simulink model "adm_pcie_9h7_dts_dual_4x100g_dsp_8b_1ant"  (R2019a)
settings: Solver=VariableStepAuto  StartTime=0.0  StopTime=10.0  RelTol=1e-3
undefined symbols (not defined in the file): datetime, fft_stages, posixtime
libraries: xbsIndex_r4 x17321, casper_library_misc x181, xps_library x11, casper_library_delays x8, casper_library_sources x8, casper_library_reorder x5, casper_library_scopes x4
(part 22 of 187)

== system adm_pcie_9h7_dts_dual_4x100g_dsp_8b_1ant/pipeline0/input/bit_stats ==
  din : Inport
  Counter1 : xbsIndex_r4/Counter  cnt_type=Free Running  cnt_to=Inf  operation=Up  start_count=0  cnt_by_val=1  arith_type=Unsigned  n_bits=20  bin_pt=0  load_pin=off  rst=off  en=off  explicit_period=on  period=1  use_behavioral_HDL=off  implementation=Fabric  use_rpm=on  dbl_ovrd=off  block_type=counter
      settings: xl_area=[0, 0, 0, 0, 0, 0, 0]
  Mux : xbsIndex_r4/Mux  inputs=32  en=off  latency=1  precision=Full  arith_type=Unsigned  n_bits=16  bin_pt=14  quantization=Truncate  overflow=Wrap  dbl_ovrd=off  block_type=mux
  Slice1 : xbsIndex_r4/Slice  nbits=1  boolean_output=on  mode=Upper Bit Location + Width  bit1=0  base1=MSB of Input  bit0=19  base0=LSB of Input  dbl_ovrd=off  block_type=slice
      settings: infoedit="Extracts a given range of bits from each input sample and presents it at the output.  The output type is ordinarily unsigned with binary point at zero, but can be Boolean when the slice is one bit wide.<P><P>Hardware notes: In hardware this block costs nothing."  block_version=10.1.3
  Slice2 : xbsIndex_r4/Slice  nbits=1  boolean_output=off  mode=Lower Bit Location + Width  bit1=0  base1=MSB of Input  bit0=5  base0=LSB of Input  dbl_ovrd=off  block_type=slice
      settings: block_version=10.1.3
  Slice3 : xbsIndex_r4/Slice  nbits=5  boolean_output=off  mode=Lower Bit Location + Width  bit1=0  base1=MSB of Input  bit0=0  base0=LSB of Input  dbl_ovrd=off  block_type=slice
      settings: block_version=10.1.3
  bus_expand1 : Subsystem  AncestorBlock=casper_library_flow_control/bus_expand  mask(bus_expand){mode=divisions of equal size, outputNum=32, outputWidth=8, outputBinaryPt=0, outputArithmeticType=0, show_format=off, outputToWorkspace=off, variablePrefix=out, outputToModelAsWell=on}
      mask prompts: outputNum "Number of outputs:"; outputWidth "Output width:"; outputBinaryPt "Output binary point position:"; outputArithmeticType "Output arithmetic type (ufix=0, fix=1, bool=2):"; show_format "Print format string?"; outputToWorkspace "Output to workspace?"; variablePrefix "Variable name prefix:"; outputToModelAsWell "Output to model as well?"
      mask help:
      | Expands a 'bus' made using a bus_create or Xilinx
      | concat block.
      | The input will be divided into the specified number
      | of outputs with the specified arithmetic types.
      | Divisions are made from most significant bit.
      mask init: same as adm_pcie_9h7_dts_dual_4x100g_dsp_8b_1ant/pipeline0/autocorr/bus_expand
      settings: AttributesFormatString=32 outputs
      mask TypeOptions mode: divisions of equal size | divisions of arbitrary size
      mask Callback mode: bus_expand_callback();
      mask Callback outputWidth: bus_expand_callback();
      mask Callback outputToWorkspace: bus_expand_callback();
  edge_detect1 : Subsystem  AncestorBlock=casper_library_misc/edge_detect  mask(edge_detect){edge=Rising, polarity=Active High, x_in=[0 0.08 0.08 0.16 0.16 0.24 0.24 0.32 0.32 0.4], y_in=[-1 -1  1  1  1  1  1  1  1  1], x_out=[0.6 0.68 0.68 0.76 0.76 0.84 0.84 0.92 0.92 1], y_out=[-1 -1  1  1 -1 -1 -1 -1 -1 -1]}
      mask prompts: edge "Edge Type"; polarity "Output Polarity"; x_in "Input X Positions"; y_in "Input Y Positions"; x_out "Output X Positions"; y_out "Output Y Positions"
      mask help: Output is active for one-cycle after each edge of the specified type (i.e. rising, falling or both).
      mask init: same as adm_pcie_9h7_dts_dual_4x100g_dsp_8b_1ant/pipeline0/corr/edge_detect
      settings: AttributesFormatString=|
      | rising edges
      | active high
      mask Help: Output is active for one-cycle after each edge of the specified type (i.e. rising, falling, or both).  Latency is zero.
      mask TypeOptions edge: Rising | Falling | Both
      mask TypeOptions polarity: Active High | Active Low
      mask Display:
      | plot(x_in_num,0.5+y_in_num*0.2);
      | plot(x_out_num,0.5+y_out_num*0.2);
  histogram : Subsystem  mask{bitwidth=8}
  input_sel : Subsystem  Tag=xps:sw_reg  AncestorBlock=xps_library/Memory/software_register  mask(swreg){io_dir=From Processor, io_delay=0, init_val=0, sample_period=1, names=reg, bitwidths=32, bin_pts=0, arith_types=0, sim_port=on, show_format=on, desc_str=|}
      mask desc_str=|
      | Input selection. The least significant 6 bits should be
      | set to ``n`` to compute the histogram for input ``n``.
      mask prompts: io_dir "I/O direction"; io_delay "I/O delay"; init_val "Initial Value"; sample_period "Sample period"; names "Bitfield names [msb...lsb]"; bitwidths "Bitfield widths"; bin_pts "Bitfield binary pts"; arith_types "Bitfield types, ufix=0, fix=1, bool=2"; sim_port "Provide sim input/output?"; show_format "Print format string?"; desc_str "Description"
      mask help: A 32-bit software-accessible register. Can be divided into bitfields of varying widths and types using the fields in the block mask.
      mask init:
      | swreg_init(gcb)
      settings: AttributesFormatString=1input:uf32.0 = 32 bits
      mask TypeOptions io_dir: To Processor | From Processor
      mask Callback io_dir:
      | mask_enables = get_param(gcb, 'MaskEnables');
      | mask_names = get_param(gcb, 'MaskNames');
      | if strcmp(get_param(gcb, 'io_dir'), 'To Processor'),
      |     mask_enables{ismember(mask_names, 'sample_period')} = 'off';
      | else
      |     mask_enables{ismember(mask_names, 'sample_period')} = 'on';
      | end
      | set_param(gcb, 'MaskEnables', mask_enables);
      mask DialogControl ParameterTabVar0 Prompt: Setup
  wires:
  [adc_hist_rst] -> histogram/2(new_acc)
  Mux/1 -> histogram/1(din)
  Counter1/1 -> Slice1/1
  Slice1/1 -> edge_detect1/1(in)
  edge_detect1/1(out) -> [adc_hist_rst]
  input_sel/1(in_reg) -> Slice3/1, Slice2/1
  Slice2/1 -> [sel_msb]
  din/1 -> bus_expand1/1(bus_in)
  Slice3/1 -> [sel_lsb]
  [sel_lsb] -> Mux/1
  bus_expand1/14(out19) -> Mux/15
  bus_expand1/7(out26) -> Mux/8
  bus_expand1/13(out20) -> Mux/14
  bus_expand1/17(out16) -> Mux/18
  bus_expand1/18(out15) -> Mux/19
  bus_expand1/11(out22) -> Mux/12
  bus_expand1/20(out13) -> Mux/21
  bus_expand1/2(out31) -> Mux/3
  bus_expand1/9(out24) -> Mux/10
  bus_expand1/3(out30) -> Mux/4
  bus_expand1/6(out27) -> Mux/7
  bus_expand1/10(out23) -> Mux/11
  bus_expand1/21(out12) -> Mux/22
  bus_expand1/16(out17) -> Mux/17
  bus_expand1/19(out14) -> Mux/20
  bus_expand1/12(out21) -> Mux/13
  bus_expand1/4(out29) -> Mux/5
  bus_expand1/1(msb_out32) -> Mux/2
  bus_expand1/15(out18) -> Mux/16
  bus_expand1/5(out28) -> Mux/6
  bus_expand1/22(out11) -> Mux/23
  bus_expand1/23(out10) -> Mux/24
  bus_expand1/24(out9) -> Mux/25
  bus_expand1/25(out8) -> Mux/26
  bus_expand1/26(out7) -> Mux/27
  bus_expand1/27(out6) -> Mux/28
  bus_expand1/28(out5) -> Mux/29
  bus_expand1/29(out4) -> Mux/30
  bus_expand1/30(out3) -> Mux/31
  bus_expand1/31(out2) -> Mux/32
  bus_expand1/32(lsb_out1) -> Mux/33
  bus_expand1/8(out25) -> Mux/9

== system adm_pcie_9h7_dts_dual_4x100g_dsp_8b_1ant/pipeline0/input/bus_mux1 ==
  sel : Inport
  d0 : Inport  Port=2
  d1 : Inport  Port=3
  d2 : Inport  Port=4
  misci : Inport  Port=5
  d_bussify : Subsystem  AncestorBlock=casper_library_flow_control/bus_create  mask(bus_create){inputNum=4}
      mask prompts: inputNum "Number of inputs:"
      mask init:
      | bus_create_init(gcb,...
      |     'inputNum', inputNum);
  dmisc : xbsIndex_r4/Delay  rst=off  infoeditControl=Selection of Reset will increase slice count due to use of real FFs and instead of SRLs  en=off  latency=1  reg_retiming=on  dbl_ovrd=off  block_type=delay
  expand0 : Subsystem  AncestorBlock=casper_library_flow_control/bus_expand  mask(bus_expand){mode=divisions of arbitrary size, outputNum=1, outputWidth=[64;64;64;64], outputBinaryPt=[0  0  0  0], outputArithmeticType=[0  0  0  0], show_format=on, outputToWorkspace=off, variablePrefix=, outputToModelAsWell=on}
      mask prompts: outputNum "Number of outputs:"; outputWidth "Output width [msb ... lsb]:"; outputBinaryPt "Output binary point position [msb ... lsb]:"; outputArithmeticType "Output arithmetic type (ufix=0, fix=1, bool=2) [msb ... lsb]:"; show_format "Print format string?"; outputToWorkspace "Output to workspace?"; variablePrefix "Variable name prefix:"; outputToModelAsWell "Output to model as well?"
      mask help:
      | Expands a 'bus' made using a bus_create or Xilinx
      | concat block.
      | The input will be divided into the specified number
      | of outputs with the specified arithmetic types.
      | Divisions are made from most significant bit.
      mask init: same as adm_pcie_9h7_dts_dual_4x100g_dsp_8b_1ant/pipeline0/autocorr/bus_expand
      settings: AttributesFormatString=4 outputs: uf64.0,uf64.0,uf64.0,uf64.0,
      mask TypeOptions mode: divisions of equal size | divisions of arbitrary size
      mask Callback mode: bus_expand_callback();
      mask Callback outputWidth: bus_expand_callback();
      mask Callback outputToWorkspace: bus_expand_callback();
  expand1 : Subsystem  AncestorBlock=casper_library_flow_control/bus_expand  mask(bus_expand){mode=divisions of arbitrary size, outputNum=1, outputWidth=[64;64;64;64], outputBinaryPt=[0  0  0  0], outputArithmeticType=[0  0  0  0], show_format=on, outputToWorkspace=off, variablePrefix=, outputToModelAsWell=on}
      mask prompts: outputNum "Number of outputs:"; outputWidth "Output width [msb ... lsb]:"; outputBinaryPt "Output binary point position [msb ... lsb]:"; outputArithmeticType "Output arithmetic type (ufix=0, fix=1, bool=2) [msb ... lsb]:"; show_format "Print format string?"; outputToWorkspace "Output to workspace?"; variablePrefix "Variable name prefix:"; outputToModelAsWell "Output to model as well?"
      mask help:
      | Expands a 'bus' made using a bus_create or Xilinx
      | concat block.
      | The input will be divided into the specified number
      | of outputs with the specified arithmetic types.
      | Divisions are made from most significant bit.
      mask init: same as adm_pcie_9h7_dts_dual_4x100g_dsp_8b_1ant/pipeline0/autocorr/bus_expand
      settings: AttributesFormatString=4 outputs: uf64.0,uf64.0,uf64.0,uf64.0,
      mask TypeOptions mode: divisions of equal size | divisions of arbitrary size
      mask Callback mode: bus_expand_callback();
      mask Callback outputWidth: bus_expand_callback();
      mask Callback outputToWorkspace: bus_expand_callback();
  expand2 : Subsystem  AncestorBlock=casper_library_flow_control/bus_expand  mask(bus_expand){mode=divisions of arbitrary size, outputNum=1, outputWidth=[64;64;64;64], outputBinaryPt=[0  0  0  0], outputArithmeticType=[0  0  0  0], show_format=on, outputToWorkspace=off, variablePrefix=, outputToModelAsWell=on}
      mask prompts: outputNum "Number of outputs:"; outputWidth "Output width [msb ... lsb]:"; outputBinaryPt "Output binary point position [msb ... lsb]:"; outputArithmeticType "Output arithmetic type (ufix=0, fix=1, bool=2) [msb ... lsb]:"; show_format "Print format string?"; outputToWorkspace "Output to workspace?"; variablePrefix "Variable name prefix:"; outputToModelAsWell "Output to model as well?"
      mask help:
      | Expands a 'bus' made using a bus_create or Xilinx
      | concat block.
      | The input will be divided into the specified number
      | of outputs with the specified arithmetic types.
      | Divisions are made from most significant bit.
      mask init: same as adm_pcie_9h7_dts_dual_4x100g_dsp_8b_1ant/pipeline0/autocorr/bus_expand
      settings: AttributesFormatString=4 outputs: uf64.0,uf64.0,uf64.0,uf64.0,
      mask TypeOptions mode: divisions of equal size | divisions of arbitrary size
      mask Callback mode: bus_expand_callback();
      mask Callback outputWidth: bus_expand_callback();
      mask Callback outputToWorkspace: bus_expand_callback();
  mux{0..3} (4 alike) : xbsIndex_r4/Mux  inputs=3  en=off  latency=1  precision=Full  arith_type=Unsigned  n_bits=16  bin_pt=14  quantization=Truncate  overflow=Wrap  dbl_ovrd=off  block_type=mux
  sel_expand : Subsystem  AncestorBlock=casper_library_flow_control/bus_expand  mask(bus_expand){mode=divisions of equal size, outputNum=4, outputWidth=2, outputBinaryPt=0, outputArithmeticType=0, show_format=on, outputToWorkspace=off, variablePrefix=, outputToModelAsWell=on}
      mask prompts: outputNum "Number of outputs:"; outputWidth "Output width:"; outputBinaryPt "Output binary point position:"; outputArithmeticType "Output arithmetic type (ufix=0, fix=1, bool=2):"; show_format "Print format string?"; outputToWorkspace "Output to workspace?"; variablePrefix "Variable name prefix:"; outputToModelAsWell "Output to model as well?"
      mask help:
      | Expands a 'bus' made using a bus_create or Xilinx
      | concat block.
      | The input will be divided into the specified number
      | of outputs with the specified arithmetic types.
      | Divisions are made from most significant bit.
      mask init: same as adm_pcie_9h7_dts_dual_4x100g_dsp_8b_1ant/pipeline0/autocorr/bus_expand
      settings: AttributesFormatString=4 outputs: uf2.0,uf2.0,uf2.0,uf2.0,
      mask TypeOptions mode: divisions of equal size | divisions of arbitrary size
      mask Callback mode: bus_expand_callback();
      mask Callback outputWidth: bus_expand_callback();
      mask Callback outputToWorkspace: bus_expand_callback();
  out : Outport
  misco : Outport  Port=2
  wires:
  sel/1 -> sel_expand/1(bus_in)
  d0/1 -> expand0/1(bus_in)
  d1/1 -> expand1/1(bus_in)
  d2/1 -> expand2/1(bus_in)
  sel_expand/1(msb_out4) -> mux0/1
  expand0/1(msb_out4) -> mux0/2
  expand1/1(msb_out4) -> mux0/3
  expand2/1(msb_out4) -> mux0/4
  sel_expand/2(out3) -> mux1/1
  expand0/2(out3) -> mux1/2
  expand1/2(out3) -> mux1/3
  expand2/2(out3) -> mux1/4
  sel_expand/3(out2) -> mux2/1
  expand0/3(out2) -> mux2/2
  expand1/3(out2) -> mux2/3
  expand2/3(out2) -> mux2/4
  sel_expand/4(lsb_out1) -> mux3/1
  expand0/4(lsb_out1) -> mux3/2
  expand1/4(lsb_out1) -> mux3/3
  expand2/4(lsb_out1) -> mux3/4
  misci/1 -> dmisc/1
  mux0/1 -> d_bussify/1(in1)
  mux1/1 -> d_bussify/2(in2)
  mux2/1 -> d_bussify/3(in3)
  mux3/1 -> d_bussify/4(in4)
  d_bussify/1(bus_out) -> out/1
  dmisc/1 -> misco/1

== system adm_pcie_9h7_dts_dual_4x100g_dsp_8b_1ant/pipeline0/input/rms ==
  note: two clocks after
      | adc_rms_rst goes high
      | the outputs are locked
  note: To provide a means for measuring the magnitude of the signals
      | coming in to each ADC channel, we have a "calc_adc_sum_sq"
      | block which uses a single multiplier, two accumulators, and two
      | regsiters to calculate the sum of 64K ADC samples and the sum
      | of squares of 64K ADC samples.  These can be used to calculate
      | the mean (aka DC offset) and standard deviation (aka RMS) of
      | the ADC inputs.
  note: The sum_sumsq values are Fix_64_0.
      | The upper 29 bits are Fix_29_0 sum of samples.
      | The lower 35 bits are UFix_35_0 sum of squares.
  note: sum,sq,sum,sq,...
  in : Inport
  Constant : Constant  Value=0
  Counter : xbsIndex_r4/Counter  cnt_type=Free Running  cnt_to=Inf  operation=Up  start_count=0  cnt_by_val=1  arith_type=Unsigned  n_bits=16  bin_pt=0  load_pin=off  rst=off  en=off  explicit_period=off  period=1  use_behavioral_HDL=off  implementation=Fabric  use_rpm=on  dbl_ovrd=off  block_type=counter
      settings: xl_area=[0, 0, 0, 0, 0, 0, 0]
  Goto Tag Visibility : GotoTagVisibility  GotoTag=adc_rms_rst
  Slice16 : xbsIndex_r4/Slice  nbits=1  boolean_output=on  mode=Upper Bit Location + Width  bit1=0  base1=MSB of Input  bit0=19  base0=LSB of Input  dbl_ovrd=off  block_type=slice
      settings: infoedit="Extracts a given range of bits from each input sample and presents it at the output.  The output type is ordinarily unsigned with binary point at zero, but can be Boolean when the slice is one bit wide.<P><P>Hardware notes: In hardware this block costs nothing."  block_version=10.1.3
  Terminator : Terminator
  bram_ctrl : Subsystem
  bus_expand : Subsystem  AncestorBlock=casper_library_flow_control/bus_expand  mask(bus_expand){mode=divisions of equal size, outputNum=32, outputWidth=8, outputBinaryPt=0, outputArithmeticType=1, show_format=off, outputToWorkspace=off, variablePrefix=out, outputToModelAsWell=on}
      mask prompts: outputNum "Number of outputs:"; outputWidth "Output width:"; outputBinaryPt "Output binary point position:"; outputArithmeticType "Output arithmetic type (ufix=0, fix=1, bool=2):"; show_format "Print format string?"; outputToWorkspace "Output to workspace?"; variablePrefix "Variable name prefix:"; outputToModelAsWell "Output to model as well?"
      mask help:
      | Expands a 'bus' made using a bus_create or Xilinx
      | concat block.
      | The input will be divided into the specified number
      | of outputs with the specified arithmetic types.
      | Divisions are made from most significant bit.
      mask init: same as adm_pcie_9h7_dts_dual_4x100g_dsp_8b_1ant/pipeline0/autocorr/bus_expand
      settings: AttributesFormatString=32 outputs
      mask TypeOptions mode: divisions of equal size | divisions of arbitrary size
      mask Callback mode: bus_expand_callback();
      mask Callback outputWidth: bus_expand_callback();
      mask Callback outputToWorkspace: bus_expand_callback();
  calc_adc_sum_sq0 : Subsystem
  calc_adc_sum_sq1 : Subsystem
  calc_adc_sum_sq10 : Subsystem
  calc_adc_sum_sq11 : Subsystem
  calc_adc_sum_sq12 : Subsystem
  calc_adc_sum_sq13 : Subsystem
  calc_adc_sum_sq14 : Subsystem
  calc_adc_sum_sq15 : Subsystem
  calc_adc_sum_sq16 : Subsystem
  calc_adc_sum_sq17 : Subsystem
  calc_adc_sum_sq18 : Subsystem
  calc_adc_sum_sq19 : Subsystem
  calc_adc_sum_sq2 : Subsystem
  calc_adc_sum_sq20 : Subsystem
  calc_adc_sum_sq21 : Subsystem
  calc_adc_sum_sq22 : Subsystem
  calc_adc_sum_sq23 : Subsystem
  calc_adc_sum_sq24 : Subsystem
  calc_adc_sum_sq25 : Subsystem
  calc_adc_sum_sq26 : Subsystem
  calc_adc_sum_sq27 : Subsystem
  calc_adc_sum_sq28 : Subsystem
  calc_adc_sum_sq29 : Subsystem
  calc_adc_sum_sq3 : Subsystem
  calc_adc_sum_sq30 : Subsystem
  calc_adc_sum_sq31 : Subsystem
  calc_adc_sum_sq4 : Subsystem
  calc_adc_sum_sq5 : Subsystem
  calc_adc_sum_sq6 : Subsystem
  calc_adc_sum_sq7 : Subsystem
  calc_adc_sum_sq8 : Subsystem
  calc_adc_sum_sq9 : Subsystem
  edge_detect : Subsystem  AncestorBlock=casper_library_misc/edge_detect  mask(edge_detect){edge=Rising, polarity=Active High, x_in=[0 0.08 0.08 0.16 0.16 0.24 0.24 0.32 0.32 0.4], y_in=[-1 -1  1  1  1  1  1  1  1  1], x_out=[0.6 0.68 0.68 0.76 0.76 0.84 0.84 0.92 0.92 1], y_out=[-1 -1  1  1 -1 -1 -1 -1 -1 -1]}
      mask prompts: edge "Edge Type"; polarity "Output Polarity"; x_in "Input X Positions"; y_in "Input Y Positions"; x_out "Output X Positions"; y_out "Output Y Positions"
      mask help: Output is active for one-cycle after each edge of the specified type (i.e. rising, falling or both).
      mask init: same as adm_pcie_9h7_dts_dual_4x100g_dsp_8b_1ant/pipeline0/corr/edge_detect
      settings: AttributesFormatString=|
      | rising edges
      | active high
      mask Help: Output is active for one-cycle after each edge of the specified type (i.e. rising, falling, or both).  Latency is zero.
      mask TypeOptions edge: Rising | Falling | Both
      mask TypeOptions polarity: Active High | Active Low
      mask Display:
      | plot(x_in_num,0.5+y_in_num*0.2);
      | plot(x_out_num,0.5+y_out_num*0.2);
  enable : Subsystem  Tag=xps:sw_reg  AncestorBlock=xps_library/Memory/software_register  mask(swreg){io_dir=From Processor, io_delay=0, init_val=0, sample_period=1, names=reg, bitwidths=32, bin_pts=0, arith_types=0, sim_port=on, show_format=off, desc_str=|}
      mask desc_str=|
      | Enable statistics recording. If the least-significant bit
      | is ``1``, statistics will be recorded to RAM.
      mask prompts: io_dir "I/O direction"; io_delay "I/O delay"; init_val "Initial Value"; sample_period "Sample period"; names "Bitfield names [msb...lsb]"; bitwidths "Bitfield widths"; bin_pts "Bitfield binary pts"; arith_types "Bitfield types, ufix=0, fix=1, bool=2"; sim_port "Provide sim input/output?"; show_format "Print format string?"; desc_str "Description"
      mask help: A 32-bit software-accessible register. Can be divided into bitfields of varying widths and types using the fields in the block mask.
      mask init:
      | swreg_init(gcb)
      settings: AttributesFormatString=1input
      mask TypeOptions io_dir: To Processor | From Processor
      mask Callback io_dir:
      | mask_enables = get_param(gcb, 'MaskEnables');
      | mask_names = get_param(gcb, 'MaskNames');
      | if strcmp(get_param(gcb, 'io_dir'), 'To Processor'),
      |     mask_enables{ismember(mask_names, 'sample_period')} = 'off';
      | else
      |     mask_enables{ismember(mask_names, 'sample_period')} = 'on';
      | end
      | set_param(gcb, 'MaskEnables', mask_enables);
      mask DialogControl ParameterTabVar0 Prompt: Setup
  levels : Subsystem  Tag=xps:bram  AncestorBlock=xps_library/Memory/shared_bram  mask{sample_rate=1, init_vals=[0:2^10-1], data_bin_pt=0, optimization=Minimum_Area, reg_core_output=on, reg_prim_output=on, data_width=64, addr_width=9, arith_type=Unsigned, desc_str=|, type_desc=uint64}
      mask desc_str=|
      | Multi-channel statistics. For the ``n`` th 64-bit word, the
      | least signficant 32 bits represent the accumulated
      | ADC power, accumulated over 65536 samples and
      | stored as an unsigned 32-bit integer.
      | The most significant 32 bits represent the sum of
      | 65536 ADC samples stored as a signed 32-bit integer.
      mask prompts: sample_rate "Sample rate"; init_vals "Initial values (simulation only)"; data_bin_pt "Data Binary Point"; reg_core_output "Register Core Output"; reg_prim_output "Register Primitive Output"; data_width "Data Width"; addr_width "Address width"; arith_type "Output Data Type"; desc_str "Description"; type_desc "Word Type Description"
      mask init:
      | shared_bram_mask;
      mask TypeOptions optimization: Minimum_Area | Low_Power
      mask TypeOptions data_width: 8 | 16 | 32 | 64 | 128
      mask TypeOptions arith_type: Unsigned | Signed  (2's comp)
      mask DialogControl Container4 Prompt: Configuration
      mask DialogControl Container10 Prompt: Documentation
  lsb : xbsIndex_r4/Slice  nbits=0  boolean_output=on  mode=Lower Bit Location + Width  bit1=0  base1=MSB of Input  bit0=0  base0=LSB of Input  dbl_ovrd=off  block_type=slice
      settings: block_version=10.1.3
  tag scope: adc_rms_rst=scoped
  wires:
  Counter/1 -> Slice16/1
  Slice16/1 -> edge_detect/1(in)
  edge_detect/1(out) -> [adc_rms_rst]
  enable/1(in_reg) -> lsb/1
  bram_ctrl/1(addr) -> levels/1(addr)
  bram_ctrl/2(data) -> levels/2(data_in)
  bram_ctrl/3(we) -> levels/3(we)
  Constant/1 -> enable/1(sim_1)
  levels/1(data_out) -> Terminator/1
  in/1 -> bus_expand/1(bus_in)
  lsb/1 -> bram_ctrl/1(en)
  bus_expand/1(msb_out32) -> calc_adc_sum_sq0/1(in)
  calc_adc_sum_sq0/1(sum_sumsq) -> bram_ctrl/2(adc0)
  bus_expand/2(out31) -> calc_adc_sum_sq1/1(in)
  bus_expand/3(out30) -> calc_adc_sum_sq2/1(in)
  bus_expand/4(out29) -> calc_adc_sum_sq3/1(in)
  bus_expand/5(out28) -> calc_adc_sum_sq4/1(in)
  bus_expand/6(out27) -> calc_adc_sum_sq5/1(in)
  bus_expand/7(out26) -> calc_adc_sum_sq6/1(in)
  bus_expand/8(out25) -> calc_adc_sum_sq7/1(in)
  bus_expand/9(out24) -> calc_adc_sum_sq8/1(in)
  bus_expand/10(out23) -> calc_adc_sum_sq9/1(in)
  bus_expand/11(out22) -> calc_adc_sum_sq10/1(in)
  bus_expand/12(out21) -> calc_adc_sum_sq11/1(in)
  bus_expand/13(out20) -> calc_adc_sum_sq12/1(in)
  bus_expand/14(out19) -> calc_adc_sum_sq13/1(in)
  bus_expand/15(out18) -> calc_adc_sum_sq14/1(in)
  bus_expand/16(out17) -> calc_adc_sum_sq15/1(in)
  bus_expand/17(out16) -> calc_adc_sum_sq16/1(in)
  bus_expand/18(out15) -> calc_adc_sum_sq17/1(in)
  bus_expand/19(out14) -> calc_adc_sum_sq24/1(in)
  bus_expand/20(out13) -> calc_adc_sum_sq25/1(in)
  bus_expand/21(out12) -> calc_adc_sum_sq26/1(in)
  bus_expand/22(out11) -> calc_adc_sum_sq27/1(in)
  bus_expand/23(out10) -> calc_adc_sum_sq28/1(in)
  bus_expand/24(out9) -> calc_adc_sum_sq29/1(in)
  bus_expand/25(out8) -> calc_adc_sum_sq30/1(in)
  bus_expand/26(out7) -> calc_adc_sum_sq31/1(in)
  bus_expand/27(out6) -> calc_adc_sum_sq18/1(in)
  bus_expand/28(out5) -> calc_adc_sum_sq19/1(in)
  bus_expand/29(out4) -> calc_adc_sum_sq20/1(in)
  bus_expand/30(out3) -> calc_adc_sum_sq21/1(in)
  bus_expand/31(out2) -> calc_adc_sum_sq22/1(in)
  bus_expand/32(lsb_out1) -> calc_adc_sum_sq23/1(in)
  calc_adc_sum_sq1/1(sum_sumsq) -> bram_ctrl/3(adc1)
  calc_adc_sum_sq2/1(sum_sumsq) -> bram_ctrl/4(adc2)
  calc_adc_sum_sq3/1(sum_sumsq) -> bram_ctrl/5(adc3)
  calc_adc_sum_sq4/1(sum_sumsq) -> bram_ctrl/6(adc4)
  calc_adc_sum_sq6/1(sum_sumsq) -> bram_ctrl/8(adc6)
  calc_adc_sum_sq7/1(sum_sumsq) -> bram_ctrl/9(adc7)
  calc_adc_sum_sq5/1(sum_sumsq) -> bram_ctrl/7(adc5)
  calc_adc_sum_sq9/1(sum_sumsq) -> bram_ctrl/11(adc9)
  calc_adc_sum_sq13/1(sum_sumsq) -> bram_ctrl/15(adc13)
  calc_adc_sum_sq15/1(sum_sumsq) -> bram_ctrl/17(adc15)
  calc_adc_sum_sq11/1(sum_sumsq) -> bram_ctrl/13(adc11)
  calc_adc_sum_sq14/1(sum_sumsq) -> bram_ctrl/16(adc14)
  calc_adc_sum_sq10/1(sum_sumsq) -> bram_ctrl/12(adc10)
  calc_adc_sum_sq12/1(sum_sumsq) -> bram_ctrl/14(adc12)
  calc_adc_sum_sq8/1(sum_sumsq) -> bram_ctrl/10(adc8)
  calc_adc_sum_sq17/1(sum_sumsq) -> bram_ctrl/19(adc17)
  calc_adc_sum_sq18/1(sum_sumsq) -> bram_ctrl/28(adc26)
  calc_adc_sum_sq19/1(sum_sumsq) -> bram_ctrl/29(adc27)
  calc_adc_sum_sq20/1(sum_sumsq) -> bram_ctrl/30(adc28)
  calc_adc_sum_sq21/1(sum_sumsq) -> bram_ctrl/31(adc29)
  calc_adc_sum_sq22/1(sum_sumsq) -> bram_ctrl/32(adc30)
  calc_adc_sum_sq23/1(sum_sumsq) -> bram_ctrl/33(adc31)
  calc_adc_sum_sq24/1(sum_sumsq) -> bram_ctrl/20(adc18)
  calc_adc_sum_sq25/1(sum_sumsq) -> bram_ctrl/21(adc19)
  calc_adc_sum_sq26/1(sum_sumsq) -> bram_ctrl/22(adc20)
  calc_adc_sum_sq27/1(sum_sumsq) -> bram_ctrl/23(adc21)
  calc_adc_sum_sq28/1(sum_sumsq) -> bram_ctrl/24(adc22)
  calc_adc_sum_sq30/1(sum_sumsq) -> bram_ctrl/26(adc24)
  calc_adc_sum_sq31/1(sum_sumsq) -> bram_ctrl/27(adc25)
  calc_adc_sum_sq16/1(sum_sumsq) -> bram_ctrl/18(adc16)
  calc_adc_sum_sq29/1(sum_sumsq) -> bram_ctrl/25(adc23)

== system adm_pcie_9h7_dts_dual_4x100g_dsp_8b_1ant/pipeline0/input/source_sel0 ==
  sim_1 : Inport
  adm_pcie_9h7_dts_dual_4x100g_dsp_8b_1ant_pipeline0_input_source_sel0_user_data_out : xbsIndex_r4/Gateway In  gui_display_data_type=Fixed-point  arith_type=Unsigned  n_bits=32  bin_pt=0  preci_type=Single  exp_width=8  frac_width=24  rows=1  columns=1  quantization="Round  (unbiased: +/- Inf)"  overflow=Saturate  period=1  UseAsADC=off  ADCChannel='1'  interface=None  automatic_assignment=on  address_offset=hex2dec('00')  intf_name=''  intf_description=''  default_value=0  timing_constraint=None  locs_specified=off  LOCs={}  io_standard={}  inherit_from_input=off  hdl_port=on  dbl_ovrd=off  block_type=gatewayin
  convert1_1 : DataTypeConversion  OutDataTypeStr=fixdt('ufix32_En0')  LockScale=on
  convert2_1 : DataTypeConversion  OutDataTypeStr=fixdt('ufix32_En0')  ConvertRealWorld=Stored Integer (SI)  LockScale=on
  gain_1 : Gain
  io_delay : xbsIndex_r4/Delay  rst=off  infoeditControl=Selection of Reset will increase slice count due to use of real FFs and instead of SRLs  en=off  latency=0  reg_retiming=on  dbl_ovrd=off  block_type=delay
  reint1 : xbsIndex_r4/Reinterpret  force_arith_type=on  arith_type=Unsigned  force_bin_pt=on  bin_pt=0  block_type=reinterpret
  slice_reg : xbsIndex_r4/Slice  nbits=32  boolean_output=off  mode=Lower Bit Location + Width  bit1=0  base1=MSB of Input  bit0=0  base0=LSB of Input  dbl_ovrd=off  block_type=slice
  in_reg : Outport
  wires:
  adm_pcie_9h7_dts_dual_4x100g_dsp_8b_1ant_pipeline0_input_source_sel0_user_data_out/1 -> io_delay/1
  sim_1/1 -> convert1_1/1
  convert1_1/1 -> convert2_1/1
  convert2_1/1 -> gain_1/1
  gain_1/1 -> adm_pcie_9h7_dts_dual_4x100g_dsp_8b_1ant_pipeline0_input_source_sel0_user_data_out/1
  io_delay/1 -> slice_reg/1
  slice_reg/1 -> reint1/1
  reint1/1 -> in_reg/1

== system adm_pcie_9h7_dts_dual_4x100g_dsp_8b_1ant/pipeline0/lo/0 ==
  sync : Inport
  rst : Inport  Port=2
  din0 : Inport  Port=3
  din1 : Inport  Port=4
  din2 : Inport  Port=5
  din3 : Inport  Port=6
  din4 : Inport  Port=7
  din5 : Inport  Port=8
  din6 : Inport  Port=9
  din7 : Inport  Port=10
  0 : Subsystem
  1 : Subsystem
  2 : Subsystem
  3 : Subsystem
  4 : Subsystem
  5 : Subsystem
  6 : Subsystem
  7 : Subsystem
  CMult : xbsIndex_r4/CMult  const=0  gui_display_data_type=Fixed-point  const_n_bits=4  const_bin_pt=0  float_type=Single  exp_bits=8  fraction_bits=24  en=off  latency=1  precision=User Defined  arith_type="Signed  (2's comp)"  n_bits=phase_bits + parallel_bits  bin_pt=phase_bits-1  quantization=Truncate  overflow=Wrap  use_behavioral_HDL=on  mem_type=Distributed RAM  pipeline=off  dbl_ovrd=off  block_type=cmult
  CMult1 : xbsIndex_r4/CMult  const=1  gui_display_data_type=Fixed-point  const_n_bits=4  const_bin_pt=0  float_type=Single  exp_bits=8  fraction_bits=24  en=off  latency=1  precision=User Defined  arith_type="Signed  (2's comp)"  n_bits=phase_bits + parallel_bits  bin_pt=phase_bits-1  quantization=Truncate  overflow=Wrap  use_behavioral_HDL=on  mem_type=Distributed RAM  pipeline=off  dbl_ovrd=off  block_type=cmult
  CMult2 : xbsIndex_r4/CMult  const=2  gui_display_data_type=Fixed-point  const_n_bits=4  const_bin_pt=0  float_type=Single  exp_bits=8  fraction_bits=24  en=off  latency=1  precision=User Defined  arith_type="Signed  (2's comp)"  n_bits=phase_bits + parallel_bits  bin_pt=phase_bits-1  quantization=Truncate  overflow=Wrap  use_behavioral_HDL=on  mem_type=Distributed RAM  pipeline=off  dbl_ovrd=off  block_type=cmult
  CMult3 : xbsIndex_r4/CMult  const=3  gui_display_data_type=Fixed-point  const_n_bits=4  const_bin_pt=0  float_type=Single  exp_bits=8  fraction_bits=24  en=off  latency=1  precision=User Defined  arith_type="Signed  (2's comp)"  n_bits=phase_bits + parallel_bits  bin_pt=phase_bits-1  quantization=Truncate  overflow=Wrap  use_behavioral_HDL=on  mem_type=Distributed RAM  pipeline=off  dbl_ovrd=off  block_type=cmult
  CMult4 : xbsIndex_r4/CMult  const=4  gui_display_data_type=Fixed-point  const_n_bits=4  const_bin_pt=0  float_type=Single  exp_bits=8  fraction_bits=24  en=off  latency=1  precision=User Defined  arith_type="Signed  (2's comp)"  n_bits=phase_bits + parallel_bits  bin_pt=phase_bits-1  quantization=Truncate  overflow=Wrap  use_behavioral_HDL=on  mem_type=Distributed RAM  pipeline=off  dbl_ovrd=off  block_type=cmult
  CMult5 : xbsIndex_r4/CMult  const=5  gui_display_data_type=Fixed-point  const_n_bits=4  const_bin_pt=0  float_type=Single  exp_bits=8  fraction_bits=24  en=off  latency=1  precision=User Defined  arith_type="Signed  (2's comp)"  n_bits=phase_bits + parallel_bits  bin_pt=phase_bits-1  quantization=Truncate  overflow=Wrap  use_behavioral_HDL=on  mem_type=Distributed RAM  pipeline=off  dbl_ovrd=off  block_type=cmult
  CMult6 : xbsIndex_r4/CMult  const=6  gui_display_data_type=Fixed-point  const_n_bits=4  const_bin_pt=0  float_type=Single  exp_bits=8  fraction_bits=24  en=off  latency=1  precision=User Defined  arith_type="Signed  (2's comp)"  n_bits=phase_bits + parallel_bits  bin_pt=phase_bits-1  quantization=Truncate  overflow=Wrap  use_behavioral_HDL=on  mem_type=Distributed RAM  pipeline=off  dbl_ovrd=off  block_type=cmult
  CMult7 : xbsIndex_r4/CMult  const=7  gui_display_data_type=Fixed-point  const_n_bits=4  const_bin_pt=0  float_type=Single  exp_bits=8  fraction_bits=24  en=off  latency=1  precision=User Defined  arith_type="Signed  (2's comp)"  n_bits=phase_bits + parallel_bits  bin_pt=phase_bits-1  quantization=Truncate  overflow=Wrap  use_behavioral_HDL=on  mem_type=Distributed RAM  pipeline=off  dbl_ovrd=off  block_type=cmult
  CMult8 : xbsIndex_r4/CMult  const=8  gui_display_data_type=Fixed-point  const_n_bits=4  const_bin_pt=0  float_type=Single  exp_bits=8  fraction_bits=24  en=off  latency=0  precision=User Defined  arith_type="Signed  (2's comp)"  n_bits=phase_bits + parallel_bits  bin_pt=phase_bits-1  quantization=Truncate  overflow=Wrap  use_behavioral_HDL=on  mem_type=Distributed RAM  pipeline=off  dbl_ovrd=off  block_type=cmult
  Concat : xbsIndex_r4/Concat  num_inputs=2  dbl_ovrd=off  block_type=concat
  Delay : xbsIndex_r4/Delay  rst=off  infoeditControl=Selection of Reset will increase slice count due to use of real FFs and instead of SRLs  en=off  latency=8  reg_retiming=on  dbl_ovrd=off  block_type=delay
  Delay{1..25} (25 alike) : xbsIndex_r4/Delay  rst=off  infoeditControl=Selection of Reset will increase slice count due to use of real FFs and instead of SRLs  en=off  latency=1  reg_retiming=on  dbl_ovrd=off  block_type=delay
  Reinterpret : xbsIndex_r4/Reinterpret  force_arith_type=on  arith_type="Signed  (2's comp)"  force_bin_pt=on  bin_pt=phase_bits - 1  block_type=reinterpret
  Slice : xbsIndex_r4/Slice  nbits=phase_bits  boolean_output=off  mode=Lower Bit Location + Width  bit1=0  base1=MSB of Input  bit0=0  base0=LSB of Input  dbl_ovrd=off  block_type=slice
  phase_offset_lsb : Subsystem  Tag=xps:sw_reg  AncestorBlock=xps_library/Memory/software_register  mask(swreg){io_dir=From Processor, io_delay=0, init_val=0, sample_period=1, names=reg, bitwidths=32, bin_pts=0, arith_types=0, sim_port=on, show_format=on}
      mask prompts: io_dir "I/O direction"; io_delay "I/O delay"; init_val "Initial Value"; sample_period "Sample period"; names "Bitfield names [msb...lsb]"; bitwidths "Bitfield widths"; bin_pts "Bitfield binary pts"; arith_types "Bitfield types, ufix=0, fix=1, bool=2"; sim_port "Provide sim input/output?"; show_format "Print format string?"
      mask help: A 32-bit software-accessible register. Can be divided into bitfields of varying widths and types using the fields in the block mask.
      mask init:
      | swreg_init(gcb)
      settings: AttributesFormatString=1input:uf32.0 = 32 bits
      mask TypeOptions io_dir: To Processor | From Processor
      mask Callback io_dir:
      | mask_enables = get_param(gcb, 'MaskEnables');
      | mask_names = get_param(gcb, 'MaskNames');
      | if strcmp(get_param(gcb, 'io_dir'), 'To Processor'),
      |     mask_enables{ismember(mask_names, 'sample_period')} = 'off';
      | else
      |     mask_enables{ismember(mask_names, 'sample_period')} = 'on';
      | end
      | set_param(gcb, 'MaskEnables', mask_enables);
      mask DialogControl ParameterTabVar0 Prompt: Setup
  phase_offset_msb : Subsystem  Tag=xps:sw_reg  AncestorBlock=xps_library/Memory/software_register  mask(swreg){io_dir=From Processor, io_delay=0, init_val=0, sample_period=1, names=reg, bitwidths=32, bin_pts=0, arith_types=0, sim_port=on, show_format=on}
      mask prompts: io_dir "I/O direction"; io_delay "I/O delay"; init_val "Initial Value"; sample_period "Sample period"; names "Bitfield names [msb...lsb]"; bitwidths "Bitfield widths"; bin_pts "Bitfield binary pts"; arith_types "Bitfield types, ufix=0, fix=1, bool=2"; sim_port "Provide sim input/output?"; show_format "Print format string?"
      mask help: A 32-bit software-accessible register. Can be divided into bitfields of varying widths and types using the fields in the block mask.
      mask init:
      | swreg_init(gcb)
      settings: AttributesFormatString=1input:uf32.0 = 32 bits
      mask TypeOptions io_dir: To Processor | From Processor
      mask Callback io_dir:
      | mask_enables = get_param(gcb, 'MaskEnables');
      | mask_names = get_param(gcb, 'MaskNames');
      | if strcmp(get_param(gcb, 'io_dir'), 'To Processor'),
      |     mask_enables{ismember(mask_names, 'sample_period')} = 'off';
      | else
      |     mask_enables{ismember(mask_names, 'sample_period')} = 'on';
      | end
      | set_param(gcb, 'MaskEnables', mask_enables);
      mask DialogControl ParameterTabVar0 Prompt: Setup
  ri_to_c{,1..7} (8 alike) : casper_library_misc/ri_to_c
      settings: SourceProductName=CASPER DSP Blockset
  sync_out : Outport
  dout0 : Outport  Port=2
  dout1 : Outport  Port=3
  dout2 : Outport  Port=4
  dout3 : Outport  Port=5
  dout4 : Outport  Port=6
  dout5 : Outport  Port=7
  dout6 : Outport  Port=8
  dout7 : Outport  Port=9
  wires:
  din0/1 -> Delay3/1
  sync/1 -> Delay1/1
  0/2(dout_i) -> ri_to_c/2
  0/1(dout_r) -> ri_to_c/1
  ri_to_c/1 -> dout0/1
  Delay/1 -> sync_out/1
  [rst] -> Delay2/1
  [step] -> Delay4/1
  [offset] -> CMult/1
  CMult/1 -> 0/4(offset)
  Delay1/1 -> Delay/1
  Delay2/1 -> 0/1(rst)
  Delay3/1 -> 0/2(din)
  Delay4/1 -> 0/3(phase_step)
  Delay7/1 -> 1/3(phase_step)
  Delay6/1 -> 1/2(din)
  Delay5/1 -> 1/1(rst)
  CMult1/1 -> 1/4(offset)
  [offset] -> CMult1/1
  [step] -> Delay7/1
  [rst] -> Delay5/1
  ri_to_c1/1 -> dout1/1
  1/1(dout_r) -> ri_to_c1/1
  1/2(dout_i) -> ri_to_c1/2
  din1/1 -> Delay6/1
  din2/1 -> Delay9/1
  2/2(dout_i) -> ri_to_c2/2
  2/1(dout_r) -> ri_to_c2/1
  ri_to_c2/1 -> dout2/1
  [rst] -> Delay8/1
  [step] -> Delay10/1
  [offset] -> CMult2/1
  CMult2/1 -> 2/4(offset)
  Delay8/1 -> 2/1(rst)
  Delay9/1 -> 2/2(din)
  Delay10/1 -> 2/3(phase_step)
  Delay11/1 -> 3/3(phase_step)
  Delay13/1 -> 3/2(din)
  Delay12/1 -> 3/1(rst)
  CMult3/1 -> 3/4(offset)
  [offset] -> CMult3/1
  [step] -> Delay11/1
  [rst] -> Delay12/1
  ri_to_c3/1 -> dout3/1
  3/1(dout_r) -> ri_to_c3/1
  3/2(dout_i) -> ri_to_c3/2
  din3/1 -> Delay13/1
  din7/1 -> Delay17/1
  7/2(dout_i) -> ri_to_c7/2
  7/1(dout_r) -> ri_to_c7/1
  ri_to_c7/1 -> dout7/1
  [rst] -> Delay16/1
  [step] -> Delay15/1
  [offset] -> CMult7/1
  CMult7/1 -> 7/4(offset)
  Delay16/1 -> 7/1(rst)
  Delay17/1 -> 7/2(din)
  Delay15/1 -> 7/3(phase_step)
  Delay14/1 -> 6/3(phase_step)
  Delay25/1 -> 6/2(din)
  Delay24/1 -> 6/1(rst)
  CMult6/1 -> 6/4(offset)
  [offset] -> CMult6/1
  [step] -> Delay14/1
  [rst] -> Delay24/1
  ri_to_c6/1 -> dout6/1
  6/1(dout_r) -> ri_to_c6/1
  6/2(dout_i) -> ri_to_c6/2
  din6/1 -> Delay25/1
  din5/1 -> Delay22/1
  5/2(dout_i) -> ri_to_c5/2
  5/1(dout_r) -> ri_to_c5/1
  ri_to_c5/1 -> dout5/1
  [rst] -> Delay21/1
  [step] -> Delay23/1
  [offset] -> CMult5/1
  CMult5/1 -> 5/4(offset)
  Delay21/1 -> 5/1(rst)
  Delay22/1 -> 5/2(din)
  Delay23/1 -> 5/3(phase_step)
  Delay20/1 -> 4/3(phase_step)
  Delay19/1 -> 4/2(din)
  Delay18/1 -> 4/1(rst)
  CMult4/1 -> 4/4(offset)
  [offset] -> CMult4/1
  [step] -> Delay20/1
  [rst] -> Delay18/1
  ri_to_c4/1 -> dout4/1
  4/1(dout_r) -> ri_to_c4/1
  4/2(dout_i) -> ri_to_c4/2
  din4/1 -> Delay19/1
  rst/1 -> [rst]
  CMult8/1 -> [step]
  phase_offset_msb/1(in_reg) -> Concat/1
  phase_offset_lsb/1(in_reg) -> Concat/2
  Concat/1 -> Slice/1
  Slice/1 -> Reinterpret/1
  Reinterpret/1 -> CMult8/1, [offset]

== system adm_pcie_9h7_dts_dual_4x100g_dsp_8b_1ant/pipeline0/lo/1 ==
  sync : Inport
  rst : Inport  Port=2
  din0 : Inport  Port=3
  din1 : Inport  Port=4
  din2 : Inport  Port=5
  din3 : Inport  Port=6
  din4 : Inport  Port=7
  din5 : Inport  Port=8
  din6 : Inport  Port=9
  din7 : Inport  Port=10
  0 : Subsystem
  1 : Subsystem
  2 : Subsystem
  3 : Subsystem
  4 : Subsystem
  5 : Subsystem
  6 : Subsystem
  7 : Subsystem
  CMult : xbsIndex_r4/CMult  const=0  gui_display_data_type=Fixed-point  const_n_bits=4  const_bin_pt=0  float_type=Single  exp_bits=8  fraction_bits=24  en=off  latency=1  precision=User Defined  arith_type="Signed  (2's comp)"  n_bits=phase_bits + parallel_bits  bin_pt=phase_bits-1  quantization=Truncate  overflow=Wrap  use_behavioral_HDL=on  mem_type=Distributed RAM  pipeline=off  dbl_ovrd=off  block_type=cmult
  CMult1 : xbsIndex_r4/CMult  const=1  gui_display_data_type=Fixed-point  const_n_bits=4  const_bin_pt=0  float_type=Single  exp_bits=8  fraction_bits=24  en=off  latency=1  precision=User Defined  arith_type="Signed  (2's comp)"  n_bits=phase_bits + parallel_bits  bin_pt=phase_bits-1  quantization=Truncate  overflow=Wrap  use_behavioral_HDL=on  mem_type=Distributed RAM  pipeline=off  dbl_ovrd=off  block_type=cmult
  CMult2 : xbsIndex_r4/CMult  const=2  gui_display_data_type=Fixed-point  const_n_bits=4  const_bin_pt=0  float_type=Single  exp_bits=8  fraction_bits=24  en=off  latency=1  precision=User Defined  arith_type="Signed  (2's comp)"  n_bits=phase_bits + parallel_bits  bin_pt=phase_bits-1  quantization=Truncate  overflow=Wrap  use_behavioral_HDL=on  mem_type=Distributed RAM  pipeline=off  dbl_ovrd=off  block_type=cmult
  CMult3 : xbsIndex_r4/CMult  const=3  gui_display_data_type=Fixed-point  const_n_bits=4  const_bin_pt=0  float_type=Single  exp_bits=8  fraction_bits=24  en=off  latency=1  precision=User Defined  arith_type="Signed  (2's comp)"  n_bits=phase_bits + parallel_bits  bin_pt=phase_bits-1  quantization=Truncate  overflow=Wrap  use_behavioral_HDL=on  mem_type=Distributed RAM  pipeline=off  dbl_ovrd=off  block_type=cmult
  CMult4 : xbsIndex_r4/CMult  const=4  gui_display_data_type=Fixed-point  const_n_bits=4  const_bin_pt=0  float_type=Single  exp_bits=8  fraction_bits=24  en=off  latency=1  precision=User Defined  arith_type="Signed  (2's comp)"  n_bits=phase_bits + parallel_bits  bin_pt=phase_bits-1  quantization=Truncate  overflow=Wrap  use_behavioral_HDL=on  mem_type=Distributed RAM  pipeline=off  dbl_ovrd=off  block_type=cmult
  CMult5 : xbsIndex_r4/CMult  const=5  gui_display_data_type=Fixed-point  const_n_bits=4  const_bin_pt=0  float_type=Single  exp_bits=8  fraction_bits=24  en=off  latency=1  precision=User Defined  arith_type="Signed  (2's comp)"  n_bits=phase_bits + parallel_bits  bin_pt=phase_bits-1  quantization=Truncate  overflow=Wrap  use_behavioral_HDL=on  mem_type=Distributed RAM  pipeline=off  dbl_ovrd=off  block_type=cmult
  CMult6 : xbsIndex_r4/CMult  const=6  gui_display_data_type=Fixed-point  const_n_bits=4  const_bin_pt=0  float_type=Single  exp_bits=8  fraction_bits=24  en=off  latency=1  precision=User Defined  arith_type="Signed  (2's comp)"  n_bits=phase_bits + parallel_bits  bin_pt=phase_bits-1  quantization=Truncate  overflow=Wrap  use_behavioral_HDL=on  mem_type=Distributed RAM  pipeline=off  dbl_ovrd=off  block_type=cmult
  CMult7 : xbsIndex_r4/CMult  const=7  gui_display_data_type=Fixed-point  const_n_bits=4  const_bin_pt=0  float_type=Single  exp_bits=8  fraction_bits=24  en=off  latency=1  precision=User Defined  arith_type="Signed  (2's comp)"  n_bits=phase_bits + parallel_bits  bin_pt=phase_bits-1  quantization=Truncate  overflow=Wrap  use_behavioral_HDL=on  mem_type=Distributed RAM  pipeline=off  dbl_ovrd=off  block_type=cmult
  CMult8 : xbsIndex_r4/CMult  const=8  gui_display_data_type=Fixed-point  const_n_bits=4  const_bin_pt=0  float_type=Single  exp_bits=8  fraction_bits=24  en=off  latency=0  precision=User Defined  arith_type="Signed  (2's comp)"  n_bits=phase_bits + parallel_bits  bin_pt=phase_bits-1  quantization=Truncate  overflow=Wrap  use_behavioral_HDL=on  mem_type=Distributed RAM  pipeline=off  dbl_ovrd=off  block_type=cmult
  Concat : xbsIndex_r4/Concat  num_inputs=2  dbl_ovrd=off  block_type=concat
  Delay : xbsIndex_r4/Delay  rst=off  infoeditControl=Selection of Reset will increase slice count due to use of real FFs and instead of SRLs  en=off  latency=8  reg_retiming=on  dbl_ovrd=off  block_type=delay
  Delay{1..25} (25 alike) : xbsIndex_r4/Delay  rst=off  infoeditControl=Selection of Reset will increase slice count due to use of real FFs and instead of SRLs  en=off  latency=1  reg_retiming=on  dbl_ovrd=off  block_type=delay
  Reinterpret : xbsIndex_r4/Reinterpret  force_arith_type=on  arith_type="Signed  (2's comp)"  force_bin_pt=on  bin_pt=phase_bits - 1  block_type=reinterpret
  Slice : xbsIndex_r4/Slice  nbits=phase_bits  boolean_output=off  mode=Lower Bit Location + Width  bit1=0  base1=MSB of Input  bit0=0  base0=LSB of Input  dbl_ovrd=off  block_type=slice
  phase_offset_lsb : Subsystem  Tag=xps:sw_reg  AncestorBlock=xps_library/Memory/software_register  mask(swreg){io_dir=From Processor, io_delay=0, init_val=0, sample_period=1, names=reg, bitwidths=32, bin_pts=0, arith_types=0, sim_port=on, show_format=on}
      mask prompts: io_dir "I/O direction"; io_delay "I/O delay"; init_val "Initial Value"; sample_period "Sample period"; names "Bitfield names [msb...lsb]"; bitwidths "Bitfield widths"; bin_pts "Bitfield binary pts"; arith_types "Bitfield types, ufix=0, fix=1, bool=2"; sim_port "Provide sim input/output?"; show_format "Print format string?"
      mask help: A 32-bit software-accessible register. Can be divided into bitfields of varying widths and types using the fields in the block mask.
      mask init:
      | swreg_init(gcb)
      settings: AttributesFormatString=1input:uf32.0 = 32 bits
      mask TypeOptions io_dir: To Processor | From Processor
      mask Callback io_dir:
      | mask_enables = get_param(gcb, 'MaskEnables');
      | mask_names = get_param(gcb, 'MaskNames');
      | if strcmp(get_param(gcb, 'io_dir'), 'To Processor'),
      |     mask_enables{ismember(mask_names, 'sample_period')} = 'off';
      | else
      |     mask_enables{ismember(mask_names, 'sample_period')} = 'on';
      | end
      | set_param(gcb, 'MaskEnables', mask_enables);
      mask DialogControl ParameterTabVar0 Prompt: Setup
  phase_offset_msb : Subsystem  Tag=xps:sw_reg  AncestorBlock=xps_library/Memory/software_register  mask(swreg){io_dir=From Processor, io_delay=0, init_val=0, sample_period=1, names=reg, bitwidths=32, bin_pts=0, arith_types=0, sim_port=on, show_format=on}
      mask prompts: io_dir "I/O direction"; io_delay "I/O delay"; init_val "Initial Value"; sample_period "Sample period"; names "Bitfield names [msb...lsb]"; bitwidths "Bitfield widths"; bin_pts "Bitfield binary pts"; arith_types "Bitfield types, ufix=0, fix=1, bool=2"; sim_port "Provide sim input/output?"; show_format "Print format string?"
      mask help: A 32-bit software-accessible register. Can be divided into bitfields of varying widths and types using the fields in the block mask.
      mask init:
      | swreg_init(gcb)
      settings: AttributesFormatString=1input:uf32.0 = 32 bits
      mask TypeOptions io_dir: To Processor | From Processor
      mask Callback io_dir:
      | mask_enables = get_param(gcb, 'MaskEnables');
      | mask_names = get_param(gcb, 'MaskNames');
      | if strcmp(get_param(gcb, 'io_dir'), 'To Processor'),
      |     mask_enables{ismember(mask_names, 'sample_period')} = 'off';
      | else
      |     mask_enables{ismember(mask_names, 'sample_period')} = 'on';
      | end
      | set_param(gcb, 'MaskEnables', mask_enables);
      mask DialogControl ParameterTabVar0 Prompt: Setup
  ri_to_c{,1..7} (8 alike) : casper_library_misc/ri_to_c
      settings: SourceProductName=CASPER DSP Blockset
  sync_out : Outport
  dout0 : Outport  Port=2
  dout1 : Outport  Port=3
  dout2 : Outport  Port=4
  dout3 : Outport  Port=5
  dout4 : Outport  Port=6
  dout5 : Outport  Port=7
  dout6 : Outport  Port=8
  dout7 : Outport  Port=9
  wires:
  Reinterpret/1 -> [offset], CMult8/1
  Slice/1 -> Reinterpret/1
  Concat/1 -> Slice/1
  phase_offset_lsb/1(in_reg) -> Concat/2
  phase_offset_msb/1(in_reg) -> Concat/1
  CMult8/1 -> [step]
  rst/1 -> [rst]
  din4/1 -> Delay19/1
  4/2(dout_i) -> ri_to_c4/2
  4/1(dout_r) -> ri_to_c4/1
  ri_to_c4/1 -> dout4/1
  [rst] -> Delay18/1
  [step] -> Delay20/1
  [offset] -> CMult4/1
  CMult4/1 -> 4/4(offset)
  Delay18/1 -> 4/1(rst)
  Delay19/1 -> 4/2(din)
  Delay20/1 -> 4/3(phase_step)
  Delay23/1 -> 5/3(phase_step)
  Delay22/1 -> 5/2(din)
  Delay21/1 -> 5/1(rst)
  CMult5/1 -> 5/4(offset)
  [offset] -> CMult5/1
  [step] -> Delay23/1
  [rst] -> Delay21/1
  ri_to_c5/1 -> dout5/1
  5/1(dout_r) -> ri_to_c5/1
  5/2(dout_i) -> ri_to_c5/2
  din5/1 -> Delay22/1
  din6/1 -> Delay25/1
  6/2(dout_i) -> ri_to_c6/2
  6/1(dout_r) -> ri_to_c6/1
  ri_to_c6/1 -> dout6/1
  [rst] -> Delay24/1
  [step] -> Delay14/1
  [offset] -> CMult6/1
  CMult6/1 -> 6/4(offset)
  Delay24/1 -> 6/1(rst)
  Delay25/1 -> 6/2(din)
  Delay14/1 -> 6/3(phase_step)
  Delay15/1 -> 7/3(phase_step)
  Delay17/1 -> 7/2(din)
  Delay16/1 -> 7/1(rst)
  CMult7/1 -> 7/4(offset)
  [offset] -> CMult7/1
  [step] -> Delay15/1
  [rst] -> Delay16/1
  ri_to_c7/1 -> dout7/1
  7/1(dout_r) -> ri_to_c7/1
  7/2(dout_i) -> ri_to_c7/2
  din7/1 -> Delay17/1
  din3/1 -> Delay13/1
  3/2(dout_i) -> ri_to_c3/2
  3/1(dout_r) -> ri_to_c3/1
  ri_to_c3/1 -> dout3/1
  [rst] -> Delay12/1
  [step] -> Delay11/1
  [offset] -> CMult3/1
  CMult3/1 -> 3/4(offset)
  Delay12/1 -> 3/1(rst)
  Delay13/1 -> 3/2(din)
  Delay11/1 -> 3/3(phase_step)
  Delay10/1 -> 2/3(phase_step)
  Delay9/1 -> 2/2(din)
  Delay8/1 -> 2/1(rst)
  CMult2/1 -> 2/4(offset)
  [offset] -> CMult2/1
  [step] -> Delay10/1
  [rst] -> Delay8/1
  ri_to_c2/1 -> dout2/1
  2/1(dout_r) -> ri_to_c2/1
  2/2(dout_i) -> ri_to_c2/2
  din2/1 -> Delay9/1
  din1/1 -> Delay6/1
  1/2(dout_i) -> ri_to_c1/2
  1/1(dout_r) -> ri_to_c1/1
  ri_to_c1/1 -> dout1/1
  [rst] -> Delay5/1
  [step] -> Delay7/1
  [offset] -> CMult1/1
  CMult1/1 -> 1/4(offset)
  Delay5/1 -> 1/1(rst)
  Delay6/1 -> 1/2(din)
  Delay7/1 -> 1/3(phase_step)
  Delay4/1 -> 0/3(phase_step)
  Delay3/1 -> 0/2(din)
  Delay2/1 -> 0/1(rst)
  Delay1/1 -> Delay/1
  CMult/1 -> 0/4(offset)
  [offset] -> CMult/1
  [step] -> Delay4/1
  [rst] -> Delay2/1
  Delay/1 -> sync_out/1
  ri_to_c/1 -> dout0/1
  0/1(dout_r) -> ri_to_c/1
  0/2(dout_i) -> ri_to_c/2
  sync/1 -> Delay1/1
  din0/1 -> Delay3/1
